simulink model "Linear_Controller_Linear_Plant_Linear_Observer"  (R2025b)
settings: Solver=VariableStepAuto  StartTime=0.0  StopTime=100.0  RelTol=1e-3
undefined symbols (not defined in the file or in its folder): K, p
settings Model: Creator=chako  LastModifiedBy=chako

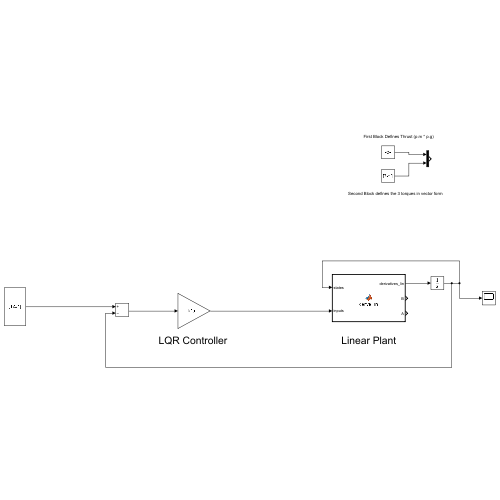
[thumbnail: Simulink's stored preview of the top-level diagram]
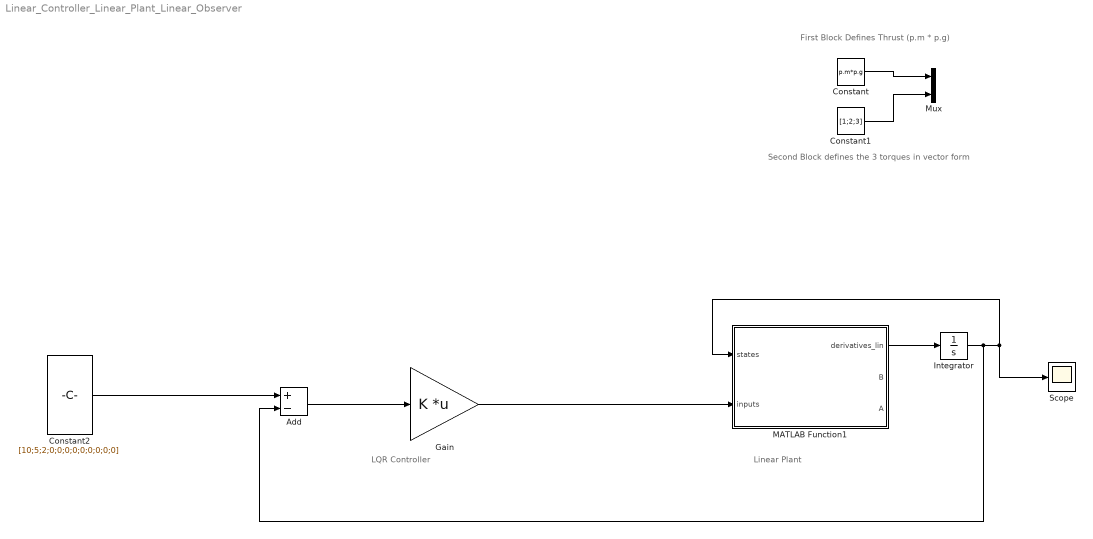
== system Linear_Controller_Linear_Plant_Linear_Observer ==
  note: Linear Plant
  note: First Block Defines Thrust (p.m * p.g)
  note: Second Block defines the 3 torques in vector form
  note: LQR Controller
  Add : Sum  Inputs=+-
  Constant : Constant  Value=p.m*p.g
  Constant1 : Constant  Value=[1;2;3]
  Constant2 : Constant  Value=[10;5;2;0;0;0;0;0;0;0;0;0]
  Gain : Gain  Gain=K  Multiplication=Matrix(K*u)
  Integrator : Integrator
  MATLAB Function1 : MATLAB Function  TreatAsAtomicUnit=on
  Mux : Mux  Inputs=2
  Scope : Scope
      settings: ActiveDisplayYMinimum=-5.4324637501756037  ActiveDisplayYMaximum=11.714719016294206
  wires:
  MATLAB Function1/1(derivatives_lin) -> Integrator/1
  Constant/1 -> Mux/1
  Constant1/1 -> Mux/2
  Gain/1 -> MATLAB Function1/2(inputs)
  Integrator/1 -> Add/2, Scope/1, MATLAB Function1/1(states)
  Constant2/1 -> Add/1
  Add/1 -> Gain/1

== matlab function Linear_Controller_Linear_Plant_Linear_Observer/MATLAB Function1 ==
  data: states input size=12; derivatives_lin output size=12; inputs input size=4; B output size=[12 4]; p parameter; A output size=[12 12]
function [derivatives_lin, B, A] = derive_lin(states, inputs, p)

    % Angles (roll, pitch, yaw) are small, approx 0
    % sin(x) = x, cos(x) = x 

    % Derivatives are zero
    % No torques (u2 to u4), but do need u1 = mg

    % eta is [phi, theta, psi] = roll pitch yaw
    xi= states(1:3); % x, y, z
    xid = states(4:6); %x_prime, y_prime, z_prime
    eta = states(7:9); % roll, pitch, yaw 
    etad = states(10:12); % roll_prime, pitch_prime, yaw_prime


    % Derivative of xi is xid

    % Calculative derivatives of xid
    % xidd = -(p.kD/p.m)*xid + [eta(2); -eta(1); 0]*p.g + [0;0;1]*inputs(1);
    % Calculative derivatives of etad
    % etadd = inputs
    A = [0 0 0   1 0 0           0 0 0   0 0 0;
         0 0 0   0 1 0           0 0 0   0 0 0;
         0 0 0   0 0 1           0 0 0   0 0 0;
         0 0 0   -p.kD/p.m 0 0   0 p.g 0   0 0 0;
         0 0 0   0 -p.kD/p.m 0   -p.g 0 0   0 0 0;
         0 0 0   0 0 -p.kD/p.m   0 0 0   0 0 0;
         0 0 0   0 0 0           0 0 0   1 0 0;
         0 0 0   0 0 0           0 0 0   0 1 0;
         0 0 0   0 0 0           0 0 0   0 0 1;
         0 0 0   0 0 0           0 0 0   0 0 0;
         0 0 0   0 0 0           0 0 0   0 0 0;
         0 0 0   0 0 0           0 0 0   0 0 0];

    B = [0 0 0 0;
         0 0 0 0;
         0 0 0 0;

         0 0 0 0;
         0 0 0 0;
         1/p.m 0 0 0;

         0 0 0 0;
         0 0 0 0;
         0 0 0 0;

         0 1/p.Ixx 0 0;
         0 0 1/p.Iyy 0;
         0 0 0 1/p.Izz;
         ];

    derivatives_lin = A * states + B * inputs;
end
